simulink model "compare_acceleration"  (R2024b)
settings: Solver=VariableStepAuto  StartTime=0.0  StopTime=10.0  RelTol=1e-3
settings Model: Creator=shohei  LastModifiedBy=shohei

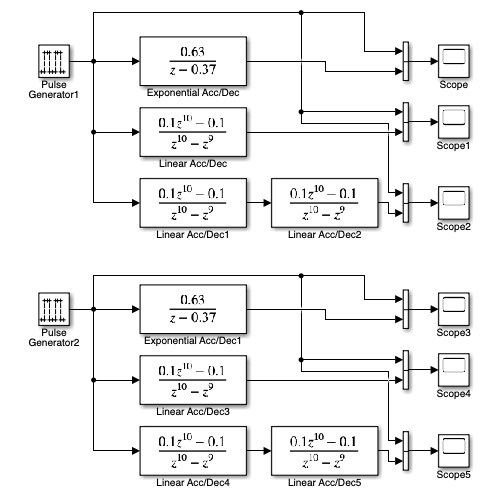
[thumbnail: Simulink's stored preview of the top-level diagram]
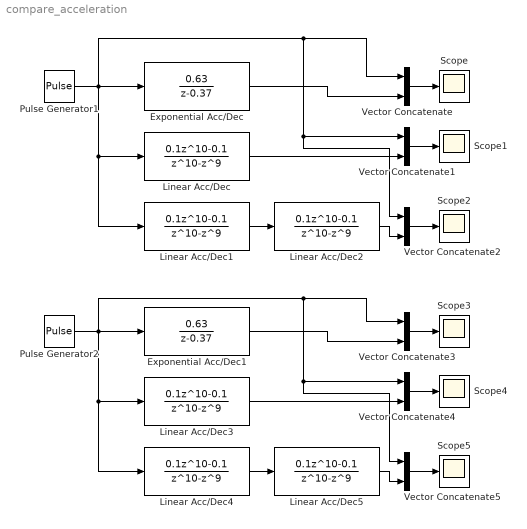
== system compare_acceleration ==
  Exponential Acc/Dec : DiscreteTransferFcn  Numerator=[0.63]  Denominator=[1 -0.37]
  Exponential Acc/Dec1 : DiscreteTransferFcn  Numerator=[0.63]  Denominator=[1 -0.37]
  Linear Acc/Dec{,1..5} (6 alike) : DiscreteTransferFcn  Numerator=[0.1 0 0 0 0 0 0 0 0 0 -0.1]  Denominator=[1 -1 0 0 0 0 0 0 0 0 0]
  Pulse Generator1 : DiscretePulseGenerator  Period=100  PulseWidth=10  SampleTime=0.05
  Pulse Generator2 : DiscretePulseGenerator  Period=100  PulseWidth=60  SampleTime=0.05
  Scope{,1..5} (6 alike) : Scope
  Vector Concatenate{,1..5} (6 alike) : Concatenate
  wires:
  Linear Acc/Dec1/1 -> Linear Acc/Dec2/1
  Pulse Generator1/1 -> Vector Concatenate2/1, Vector Concatenate1/1, Vector Concatenate/1, Linear Acc/Dec1/1, Linear Acc/Dec/1, Exponential Acc/Dec/1
  Vector Concatenate/1 -> Scope/1
  Vector Concatenate1/1 -> Scope1/1
  Vector Concatenate2/1 -> Scope2/1
  Exponential Acc/Dec/1 -> Vector Concatenate/2
  Linear Acc/Dec/1 -> Vector Concatenate1/2
  Linear Acc/Dec2/1 -> Vector Concatenate2/2
  Linear Acc/Dec5/1 -> Vector Concatenate5/2
  Linear Acc/Dec3/1 -> Vector Concatenate4/2
  Pulse Generator2/1 -> Vector Concatenate3/1, Vector Concatenate5/1, Vector Concatenate4/1, Linear Acc/Dec4/1, Linear Acc/Dec3/1, Exponential Acc/Dec1/1
  Vector Concatenate3/1 -> Scope3/1
  Linear Acc/Dec4/1 -> Linear Acc/Dec5/1
  Vector Concatenate5/1 -> Scope5/1
  Exponential Acc/Dec1/1 -> Vector Concatenate3/2
  Vector Concatenate4/1 -> Scope4/1
